simulink model "ctrl_typeBp"  (R2016b)
settings: Solver=ode45  StartTime=0.0  StopTime=10.0  RelTol=1e-3  EnableMultiTasking=on
undefined symbols (not defined in the file): Act_Mat_BF, Act_Mat_BR, Act_Mat_IM, Act_Mat_IR, Act_Mat_RM, Act_Mat_TM, gain_act_GASBF, gain_act_GASSF, gain_act_LBF, gain_act_LIM, gain_act_LTM, gain_act_PBF, gain_act_PIM, gain_act_PTM, gain_act_RBF, gain_act_RIM, gain_act_TBF, gain_act_TIM, gain_act_VBF, gain_act_VIM, gain_act_YBF, gain_act_YIM, gain_act_YTM, gain_GASBF, gain_GASSF, gain_global_LIM, gain_global_LTM, gain_LBF, gain_LIM, gain_oplev_LTM, gain_oplev_PIM, gain_oplev_PTM, gain_oplev_YIM, gain_oplev_YTM, gain_PBF, gain_PIM, gain_RBF, gain_RIM, gain_TBF, gain_TIM, gain_VBF, gain_VIM, gain_YBF, gain_YIM, Sens_Mat_OL, sys1
libraries: cstblocks x21, simulink x3
settings Model: Creator=TAMA Project  LastModifiedBy=miyo
settings DataIOCC: LimitDataPoints=on  SaveFormat=Array  SignalLoggingSaveFormat=ModelDataLogs
settings OptimizationCC: DefaultParameterBehavior=Inlined  BufferReuse=off  ExpressionDepthLimit=2147483647  LifeSpan=inf
settings DebuggingCC: UnderspecifiedInitializationDetection=Classic  MergeDetectMultiDrivingBlocksExec=none  FcnCallInpInsideContextMsg=warning  StateNameClashWarn=warning  InitInArrayFormatMsg=none  SFUnexpectedBacktrackingDiag=warning  SFNoUnconditionalDefaultTransitionDiag=warning  SFExecutionAtInitializationDiag=none
settings HardwareCC: ProdBitPerPointer=32  ProdBitPerSizeT=32  ProdBitPerPtrDiffT=32  ProdLargestAtomicFloat=None  ProdIntDivRoundTo=Undefined  ProdEndianess=Unspecified  ProdWordSize=32  ProdHWDeviceType=32-bit Generic
settings ModelReferenceCC: PropagateSignalLabelsOutOfModel=off
settings GRTTargetCC: TargetLangStandard=C89/C90 (ANSI)  GeneratePreprocessorConditionals=Disable all  CombineOutputUpdateFcns=off  GRTInterface=on
settings ConfigComp: CovMetricSettings=dw  CovHtmlReporting=on  CovSaveCumulativeToWorkspaceVar=on  CovSaveSingleToWorkspaceVar=on  CovExternalEMLEnable=off  CovSFcnEnable=off

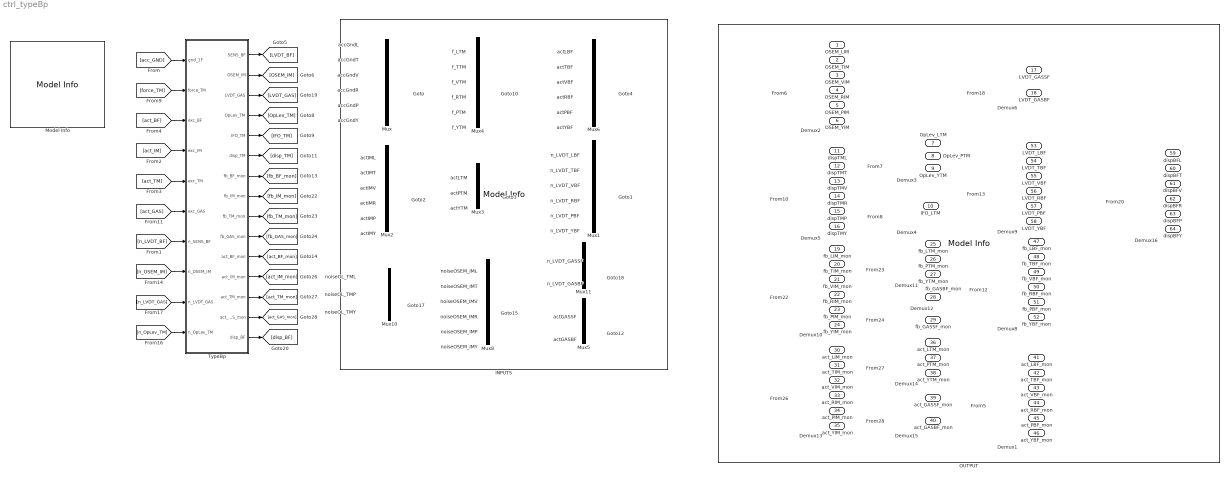
== system ctrl_typeBp ==
  accGndL : Inport
  accGndT : Inport  Port=2
  accGndV : Inport  Port=3
  accGndR : Inport  Port=4
  accGndP : Inport  Port=5
  accGndY : Inport  Port=6
  actIML : Inport  Port=7
  actIMT : Inport  Port=8
  actIMV : Inport  Port=9
  actIMR : Inport  Port=10
  actIMP : Inport  Port=11
  actIMY : Inport  Port=12
  actLTM : Inport  Port=13
  actPTM : Inport  Port=14
  actYTM : Inport  Port=15
  f_LTM : Inport  Port=16
  f_TTM : Inport  Port=17
  f_VTM : Inport  Port=18
  f_RTM : Inport  Port=19
  f_PTM : Inport  Port=20
  f_YTM : Inport  Port=21
  actGASSF : Inport  Port=22
  actGASBF : Inport  Port=23
  noiseOSEM_IML : Inport  Port=24
  noiseOSEM_IMT : Inport  Port=25
  noiseOSEM_IMV : Inport  Port=26
  noiseOSEM_IMR : Inport  Port=27
  noiseOSEM_IMP : Inport  Port=28
  noiseOSEM_IMY : Inport  Port=29
  noiseOL_TML : Inport  Port=30
  noiseOL_TMP : Inport  Port=31
  noiseOL_TMY : Inport  Port=32
  n_LVDT_GASSF : Inport  Port=33
  n_LVDT_GASBF : Inport  Port=34
  n_LVDT_LBF : Inport  Port=35
  n_LVDT_TBF : Inport  Port=36
  n_LVDT_VBF : Inport  Port=37
  n_LVDT_RBF : Inport  Port=38
  n_LVDT_PBF : Inport  Port=39
  n_LVDT_YBF : Inport  Port=40
  actLBF : Inport  Port=41
  actTBF : Inport  Port=42
  actVBF : Inport  Port=43
  actRBF : Inport  Port=44
  actPBF : Inport  Port=45
  actYBF : Inport  Port=46
  Demux{1..2,5,8..10,13,16} (8 alike) : Demux  Outputs=6
  Demux11 : Demux  Outputs=3
  Demux12 : Demux  Outputs=2
  Demux14 : Demux  Outputs=3
  Demux15 : Demux  Outputs=2
  Demux3 : Demux  Outputs=3
  Demux4 : Demux  Outputs=1
  Demux6 : Demux  Outputs=2
  INPUTS : simulink/Model-Wide Utilities/Model Info  BlockCM=none  Frame=on  DisplayStringWithTags=_  HorizontalTextAlignment=Left  LeftAlignmentValue=0.02  SourceBlockDiagram=ctrl_typeBp  TagMaxNumber=20
  Model Info : simulink/Model-Wide Utilities/Model Info  BlockCM=none  Frame=on  DisplayStringWithTags=|  HorizontalTextAlignment=Left  LeftAlignmentValue=0.02  SourceBlockDiagram=ctrl_typeBp  TagMaxNumber=20
      | [MODEL INFORMATION]
      | 
      | ModelName: %<ModelName>
      | LastUpdate : %<LastModificationDate>
      | 
      | TypeBp control model
  Mux{,1..2,4,6,8} (6 alike) : Mux  Inputs=6
  Mux10 : Mux  Inputs=3
  Mux11 : Mux  Inputs=2
  Mux3 : Mux  Inputs=3
  Mux5 : Mux  Inputs=2
  OUTPUT : simulink/Model-Wide Utilities/Model Info  BlockCM=none  Frame=on  DisplayStringWithTags=_  HorizontalTextAlignment=Left  LeftAlignmentValue=0.02  SourceBlockDiagram=ctrl_typeBp  TagMaxNumber=20
  TypeBp : Subsystem
  OSEM_LIM : Outport
  OSEM_TIM : Outport  Port=2
  OSEM_VIM : Outport  Port=3
  OSEM_RIM : Outport  Port=4
  OSEM_PIM : Outport  Port=5
  OSEM_YIM : Outport  Port=6
  OpLev_LTM : Outport  Port=7
  OpLev_PTM : Outport  Port=8
  OpLev_YTM : Outport  Port=9
  IFO_LTM : Outport  Port=10
  dispTML : Outport  Port=11
  dispTMT : Outport  Port=12
  dispTMV : Outport  Port=13
  dispTMR : Outport  Port=14
  dispTMP : Outport  Port=15
  dispTMY : Outport  Port=16
  LVDT_GASSF : Outport  Port=17
  LVDT_GASBF : Outport  Port=18
  fb_LIM_mon : Outport  Port=19
  fb_TIM_mon : Outport  Port=20
  fb_VIM_mon : Outport  Port=21
  fb_RIM_mon : Outport  Port=22
  fb_PIM_mon : Outport  Port=23
  fb_YIM_mon : Outport  Port=24
  fb_LTM_mon : Outport  Port=25
  fb_PTM_mon : Outport  Port=26
  fb_YTM_mon : Outport  Port=27
  fb_GASBF_mon : Outport  Port=28
  fb_GASSF_mon : Outport  Port=29
  act_LIM_mon : Outport  Port=30
  act_TIM_mon : Outport  Port=31
  act_VIM_mon : Outport  Port=32
  act_RIM_mon : Outport  Port=33
  act_PIM_mon : Outport  Port=34
  act_YIM_mon : Outport  Port=35
  act_LTM_mon : Outport  Port=36
  act_PTM_mon : Outport  Port=37
  act_YTM_mon : Outport  Port=38
  act_GASSF_mon : Outport  Port=39
  act_GASBF_mon : Outport  Port=40
  act_LBF_mon : Outport  Port=41
  act_TBF_mon : Outport  Port=42
  act_VBF_mon : Outport  Port=43
  act_RBF_mon : Outport  Port=44
  act_PBF_mon : Outport  Port=45
  act_YBF_mon : Outport  Port=46
  fb_LBF_mon : Outport  Port=47
  fb_TBF_mon : Outport  Port=48
  fb_VBF_mon : Outport  Port=49
  fb_RBF_mon : Outport  Port=50
  fb_PBF_mon : Outport  Port=51
  fb_YBF_mon : Outport  Port=52
  LVDT_LBF : Outport  Port=53
  LVDT_TBF : Outport  Port=54
  LVDT_VBF : Outport  Port=55
  LVDT_RBF : Outport  Port=56
  LVDT_PBF : Outport  Port=57
  LVDT_YBF : Outport  Port=58
  dispBFL : Outport  Port=59
  dispBFT : Outport  Port=60
  dispBFV : Outport  Port=61
  dispBFR : Outport  Port=62
  dispBFP : Outport  Port=63
  dispBFY : Outport  Port=64
  wires:
  accGndL/1 -> Mux/1
  accGndT/1 -> Mux/2
  accGndV/1 -> Mux/3
  accGndR/1 -> Mux/4
  accGndP/1 -> Mux/5
  accGndY/1 -> Mux/6
  Mux/1 -> [acc_GND]
  actIML/1 -> Mux2/1
  actIMT/1 -> Mux2/2
  actIMV/1 -> Mux2/3
  actIMR/1 -> Mux2/4
  actIMP/1 -> Mux2/5
  actIMY/1 -> Mux2/6
  Mux2/1 -> [act_IM]
  actLTM/1 -> Mux3/1
  actPTM/1 -> Mux3/2
  actYTM/1 -> Mux3/3
  Mux3/1 -> [act_TM]
  [OSEM_IM] -> Demux2/1
  Demux2/1 -> OSEM_LIM/1
  Demux2/2 -> OSEM_TIM/1
  Demux2/3 -> OSEM_VIM/1
  Demux2/4 -> OSEM_RIM/1
  Demux2/5 -> OSEM_PIM/1
  Demux2/6 -> OSEM_YIM/1
  [IFO_TM] -> Demux4/1
  Demux4/1 -> IFO_LTM/1
  f_LTM/1 -> Mux4/1
  f_TTM/1 -> Mux4/2
  f_VTM/1 -> Mux4/3
  Mux4/1 -> [force_TM]
  f_YTM/1 -> Mux4/6
  f_PTM/1 -> Mux4/5
  f_RTM/1 -> Mux4/4
  [disp_TM] -> Demux5/1
  Demux5/1 -> dispTML/1
  Demux5/2 -> dispTMT/1
  Demux5/3 -> dispTMV/1
  Demux5/4 -> dispTMR/1
  Demux5/5 -> dispTMP/1
  Demux5/6 -> dispTMY/1
  actGASBF/1 -> Mux5/2
  Mux5/1 -> [act_GAS]
  noiseOSEM_IML/1 -> Mux8/1
  noiseOSEM_IMT/1 -> Mux8/2
  noiseOSEM_IMV/1 -> Mux8/3
  noiseOSEM_IMR/1 -> Mux8/4
  noiseOSEM_IMP/1 -> Mux8/5
  noiseOSEM_IMY/1 -> Mux8/6
  Mux8/1 -> [n_OSEM_IM]
  Mux10/1 -> [n_OpLev_TM]
  n_LVDT_GASBF/1 -> Mux11/2
  Mux11/1 -> [n_LVDT_GAS]
  [LVDT_GAS] -> Demux6/1
  n_LVDT_GASSF/1 -> Mux11/1
  Demux6/1 -> LVDT_GASSF/1
  Demux6/2 -> LVDT_GASBF/1
  actGASSF/1 -> Mux5/1
  [fb_IM_mon] -> Demux10/1
  Demux10/1 -> fb_LIM_mon/1
  Demux10/2 -> fb_TIM_mon/1
  Demux10/3 -> fb_VIM_mon/1
  Demux10/4 -> fb_RIM_mon/1
  Demux10/5 -> fb_PIM_mon/1
  Demux10/6 -> fb_YIM_mon/1
  [fb_TM_mon] -> Demux11/1
  Demux11/1 -> fb_LTM_mon/1
  Demux11/2 -> fb_PTM_mon/1
  Demux11/3 -> fb_YTM_mon/1
  [fb_GAS_mon] -> Demux12/1
  Demux12/1 -> fb_GASBF_mon/1
  Demux12/2 -> fb_GASSF_mon/1
  [act_IM_mon] -> Demux13/1
  Demux13/1 -> act_LIM_mon/1
  Demux13/2 -> act_TIM_mon/1
  Demux13/3 -> act_VIM_mon/1
  Demux13/4 -> act_RIM_mon/1
  Demux13/5 -> act_PIM_mon/1
  Demux13/6 -> act_YIM_mon/1
  [act_TM_mon] -> Demux14/1
  Demux14/1 -> act_LTM_mon/1
  Demux14/2 -> act_PTM_mon/1
  Demux14/3 -> act_YTM_mon/1
  [act_GAS_mon] -> Demux15/1
  Demux15/1 -> act_GASSF_mon/1
  Demux15/2 -> act_GASBF_mon/1
  n_LVDT_TBF/1 -> Mux1/2
  Mux1/1 -> [n_LVDT_BF]
  n_LVDT_LBF/1 -> Mux1/1
  n_LVDT_VBF/1 -> Mux1/3
  actTBF/1 -> Mux6/2
  Mux6/1 -> [act_BF]
  actLBF/1 -> Mux6/1
  actVBF/1 -> Mux6/3
  [act_BF_mon] -> Demux1/1
  Demux1/1 -> act_LBF_mon/1
  Demux1/2 -> act_TBF_mon/1
  Demux1/3 -> act_VBF_mon/1
  [fb_BF_mon] -> Demux8/1
  Demux8/1 -> fb_LBF_mon/1
  Demux8/2 -> fb_TBF_mon/1
  Demux8/3 -> fb_VBF_mon/1
  [LVDT_BF] -> Demux9/1
  Demux9/1 -> LVDT_LBF/1
  Demux9/2 -> LVDT_TBF/1
  Demux9/3 -> LVDT_VBF/1
  [acc_GND] -> TypeBp/1(gnd_1F)
  [force_TM] -> TypeBp/2(force_TM)
  [act_BF] -> TypeBp/3(exc_BF)
  [act_IM] -> TypeBp/4(exc_IM)
  [act_TM] -> TypeBp/5(exc_TM)
  [act_GAS] -> TypeBp/6(exc_GAS)
  [n_LVDT_BF] -> TypeBp/7(n_SENS_BF)
  [n_OSEM_IM] -> TypeBp/8(n_OSEM_IM)
  [n_LVDT_GAS] -> TypeBp/9(n_LVDT_GAS)
  [n_OpLev_TM] -> TypeBp/10(n_OpLev_TM)
  TypeBp/1(SENS_BF) -> [LVDT_BF]
  TypeBp/2(OSEM_IM) -> [OSEM_IM]
  TypeBp/3(LVDT_GAS) -> [LVDT_GAS]
  TypeBp/4(OpLev_TM) -> [OpLev_TM]
  TypeBp/5(IFO_TM) -> [IFO_TM]
  TypeBp/6(disp_TM) -> [disp_TM]
  TypeBp/7(fb_BF_mon) -> [fb_BF_mon]
  TypeBp/8(fb_IM_mon) -> [fb_IM_mon]
  TypeBp/9(fb_TM_mon) -> [fb_TM_mon]
  TypeBp/10(fb_GAS_mon) -> [fb_GAS_mon]
  TypeBp/12(act_IM_mon) -> [act_IM_mon]
  TypeBp/14(act_GAS_mon) -> [act_GAS_mon]
  actRBF/1 -> Mux6/4
  actPBF/1 -> Mux6/5
  actYBF/1 -> Mux6/6
  n_LVDT_RBF/1 -> Mux1/4
  n_LVDT_PBF/1 -> Mux1/5
  n_LVDT_YBF/1 -> Mux1/6
  Demux9/4 -> LVDT_RBF/1
  Demux9/5 -> LVDT_PBF/1
  Demux9/6 -> LVDT_YBF/1
  Demux8/4 -> fb_RBF_mon/1
  Demux8/5 -> fb_PBF_mon/1
  Demux8/6 -> fb_YBF_mon/1
  Demux1/4 -> act_RBF_mon/1
  Demux1/5 -> act_PBF_mon/1
  Demux1/6 -> act_YBF_mon/1
  TypeBp/15(disp_BF) -> [disp_BF]
  [disp_BF] -> Demux16/1
  Demux16/1 -> dispBFL/1
  Demux16/2 -> dispBFT/1
  Demux16/3 -> dispBFV/1
  Demux16/4 -> dispBFR/1
  Demux16/5 -> dispBFP/1
  Demux16/6 -> dispBFY/1
  TypeBp/11(act_BF_mon) -> [act_BF_mon]
  TypeBp/13(act_TM_mon) -> [act_TM_mon]
  noiseOL_TMP/1 -> Mux10/2
  noiseOL_TML/1 -> Mux10/1
  noiseOL_TMY/1 -> Mux10/3
  Demux3/2 -> OpLev_PTM/1
  Demux3/3 -> OpLev_YTM/1
  Demux3/1 -> OpLev_LTM/1
  [OpLev_TM] -> Demux3/1

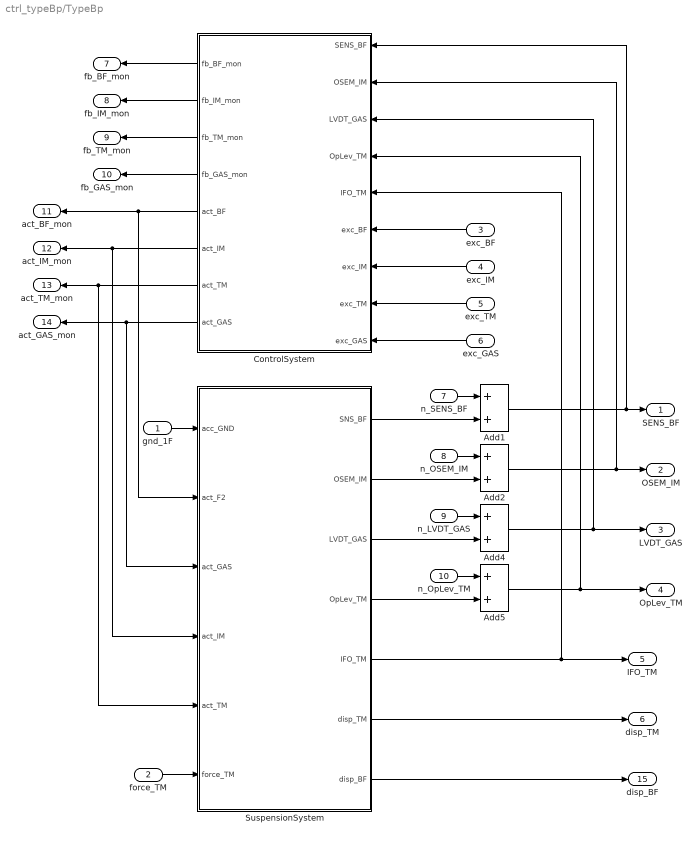
== system ctrl_typeBp/TypeBp ==
  gnd_1F : Inport
  force_TM : Inport  Port=2
  exc_BF : Inport  Port=3
  exc_IM : Inport  Port=4
  exc_TM : Inport  Port=5
  exc_GAS : Inport  Port=6
  n_SENS_BF : Inport  Port=7
  n_OSEM_IM : Inport  Port=8
  n_LVDT_GAS : Inport  Port=9
  n_OpLev_TM : Inport  Port=10
  Add{1..2,4..5} (4 alike) : Sum
  ControlSystem : Subsystem
  SuspensionSystem : Subsystem
  SENS_BF : Outport
  OSEM_IM : Outport  Port=2
  LVDT_GAS : Outport  Port=3
  OpLev_TM : Outport  Port=4
  IFO_TM : Outport  Port=5
  disp_TM : Outport  Port=6
  fb_BF_mon : Outport  Port=7
  fb_IM_mon : Outport  Port=8
  fb_TM_mon : Outport  Port=9
  fb_GAS_mon : Outport  Port=10
  act_BF_mon : Outport  Port=11
  act_IM_mon : Outport  Port=12
  act_TM_mon : Outport  Port=13
  act_GAS_mon : Outport  Port=14
  disp_BF : Outport  Port=15
  wires:
  gnd_1F/1 -> SuspensionSystem/1(acc_GND)
  force_TM/1 -> SuspensionSystem/6(force_TM)
  SuspensionSystem/6(disp_TM) -> disp_TM/1
  SuspensionSystem/2(OSEM_IM) -> Add2/2
  n_OSEM_IM/1 -> Add2/1
  SuspensionSystem/5(IFO_TM) -> IFO_TM/1, ControlSystem/5(IFO_TM)
  Add2/1 -> ControlSystem/2(OSEM_IM), OSEM_IM/1
  n_LVDT_GAS/1 -> Add4/1
  SuspensionSystem/3(LVDT_GAS) -> Add4/2
  n_OpLev_TM/1 -> Add5/1
  SuspensionSystem/4(OpLev_TM) -> Add5/2
  Add4/1 -> ControlSystem/3(LVDT_GAS), LVDT_GAS/1
  Add5/1 -> ControlSystem/4(OpLev_TM), OpLev_TM/1
  Add1/1 -> ControlSystem/1(SENS_BF), SENS_BF/1
  SuspensionSystem/1(SNS_BF) -> Add1/2
  n_SENS_BF/1 -> Add1/1
  exc_BF/1 -> ControlSystem/6(exc_BF)
  exc_IM/1 -> ControlSystem/7(exc_IM)
  exc_TM/1 -> ControlSystem/8(exc_TM)
  exc_GAS/1 -> ControlSystem/9(exc_GAS)
  ControlSystem/1(fb_BF_mon) -> fb_BF_mon/1
  ControlSystem/2(fb_IM_mon) -> fb_IM_mon/1
  ControlSystem/3(fb_TM_mon) -> fb_TM_mon/1
  ControlSystem/4(fb_GAS_mon) -> fb_GAS_mon/1
  ControlSystem/5(act_BF) -> act_BF_mon/1, SuspensionSystem/2(act_F2)
  ControlSystem/7(act_TM) -> act_TM_mon/1, SuspensionSystem/5(act_TM)
  ControlSystem/8(act_GAS) -> act_GAS_mon/1, SuspensionSystem/3(act_GAS)
  ControlSystem/6(act_IM) -> act_IM_mon/1, SuspensionSystem/4(act_IM)
  SuspensionSystem/7(disp_BF) -> disp_BF/1

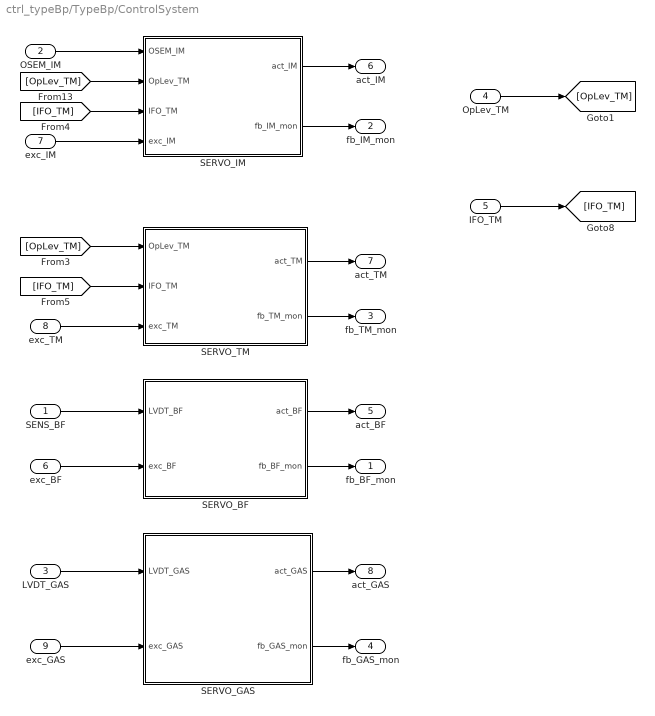
== system ctrl_typeBp/TypeBp/ControlSystem ==
  SENS_BF : Inport
  OSEM_IM : Inport  Port=2
  LVDT_GAS : Inport  Port=3
  OpLev_TM : Inport  Port=4
  IFO_TM : Inport  Port=5
  exc_BF : Inport  Port=6
  exc_IM : Inport  Port=7
  exc_TM : Inport  Port=8
  exc_GAS : Inport  Port=9
  SERVO_BF : Subsystem
  SERVO_GAS : Subsystem
  SERVO_IM : Subsystem
  SERVO_TM : Subsystem
  fb_BF_mon : Outport
  fb_IM_mon : Outport  Port=2
  fb_TM_mon : Outport  Port=3
  fb_GAS_mon : Outport  Port=4
  act_BF : Outport  Port=5
  act_IM : Outport  Port=6
  act_TM : Outport  Port=7
  act_GAS : Outport  Port=8
  wires:
  IFO_TM/1 -> [IFO_TM]
  OpLev_TM/1 -> [OpLev_TM]
  SERVO_IM/1(act_IM) -> act_IM/1
  OSEM_IM/1 -> SERVO_IM/1(OSEM_IM)
  SERVO_TM/1(act_TM) -> act_TM/1
  [OpLev_TM] -> SERVO_IM/2(OpLev_TM)
  [OpLev_TM] -> SERVO_TM/1(OpLev_TM)
  [IFO_TM] -> SERVO_IM/3(IFO_TM)
  [IFO_TM] -> SERVO_TM/2(IFO_TM)
  exc_IM/1 -> SERVO_IM/4(exc_IM)
  exc_TM/1 -> SERVO_TM/3(exc_TM)
  SERVO_IM/2(fb_IM_mon) -> fb_IM_mon/1
  SERVO_TM/2(fb_TM_mon) -> fb_TM_mon/1
  exc_GAS/1 -> SERVO_GAS/2(exc_GAS)
  SERVO_GAS/2(fb_GAS_mon) -> fb_GAS_mon/1
  LVDT_GAS/1 -> SERVO_GAS/1(LVDT_GAS)
  SERVO_GAS/1(act_GAS) -> act_GAS/1
  SENS_BF/1 -> SERVO_BF/1(LVDT_BF)
  SERVO_BF/1(act_BF) -> act_BF/1
  exc_BF/1 -> SERVO_BF/2(exc_BF)
  SERVO_BF/2(fb_BF_mon) -> fb_BF_mon/1

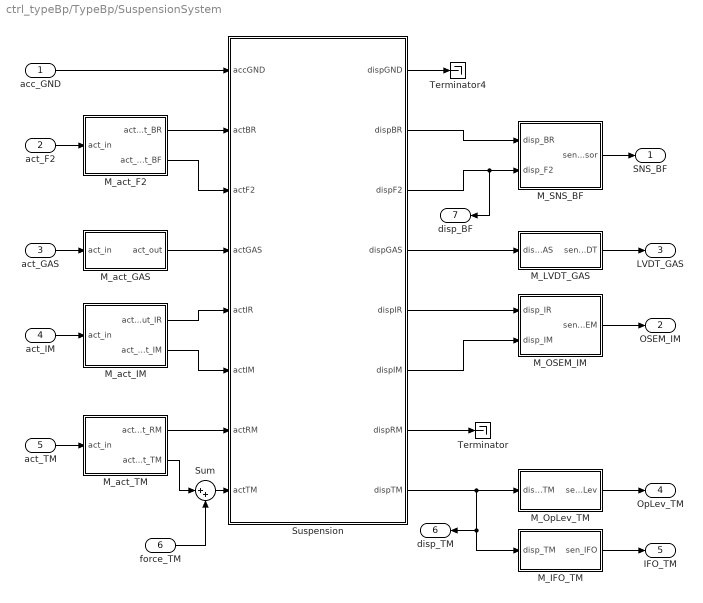
== system ctrl_typeBp/TypeBp/SuspensionSystem ==
  acc_GND : Inport
  act_F2 : Inport  Port=2
  act_GAS : Inport  Port=3
  act_IM : Inport  Port=4
  act_TM : Inport  Port=5
  force_TM : Inport  Port=6
  M_IFO_TM : Subsystem
  M_LVDT_GAS : Subsystem
  M_OSEM_IM : Subsystem
  M_OpLev_TM : Subsystem
  M_SNS_BF : Subsystem
  M_act_F2 : Subsystem
  M_act_GAS : Subsystem
  M_act_IM : Subsystem
  M_act_TM : Subsystem
  Sum : Sum  Inputs=|++
  Suspension : Subsystem
  Terminator : Terminator
  Terminator4 : Terminator
  SNS_BF : Outport
  OSEM_IM : Outport  Port=2
  LVDT_GAS : Outport  Port=3
  OpLev_TM : Outport  Port=4
  IFO_TM : Outport  Port=5
  disp_TM : Outport  Port=6
  disp_BF : Outport  Port=7
  wires:
  act_IM/1 -> M_act_IM/1(act_in)
  act_TM/1 -> M_act_TM/1(act_in)
  act_GAS/1 -> M_act_GAS/1(act_in)
  M_OSEM_IM/1(sen_OSEM) -> OSEM_IM/1
  M_LVDT_GAS/1(sen_LVDT) -> LVDT_GAS/1
  M_IFO_TM/1(sen_IFO) -> IFO_TM/1
  M_OpLev_TM/1(sen_OpLev) -> OpLev_TM/1
  act_F2/1 -> M_act_F2/1(act_in)
  acc_GND/1 -> Suspension/1(accGND)
  M_act_F2/1(act_out_BR) -> Suspension/2(actBR)
  M_act_F2/2(act_out_BF) -> Suspension/3(actF2)
  M_act_GAS/1(act_out) -> Suspension/4(actGAS)
  M_act_IM/1(act_out_IR) -> Suspension/5(actIR)
  M_act_IM/2(act_out_IM) -> Suspension/6(actIM)
  M_act_TM/1(act_out_RM) -> Suspension/7(actRM)
  M_act_TM/2(act_out_TM) -> Sum/1
  force_TM/1 -> Sum/2
  Sum/1 -> Suspension/8(actTM)
  M_SNS_BF/1(sen_F2sensor) -> SNS_BF/1
  Suspension/2(dispBR) -> M_SNS_BF/1(disp_BR)
  Suspension/3(dispF2) -> disp_BF/1, M_SNS_BF/2(disp_F2)
  Suspension/1(dispGND) -> Terminator4/1
  Suspension/4(dispGAS) -> M_LVDT_GAS/1(disp_GAS)
  Suspension/5(dispIR) -> M_OSEM_IM/1(disp_IR)
  Suspension/6(dispIM) -> M_OSEM_IM/2(disp_IM)
  Suspension/8(dispTM) -> M_IFO_TM/1(disp_TM), disp_TM/1, M_OpLev_TM/1(disp_TM)
  Suspension/7(dispRM) -> Terminator/1

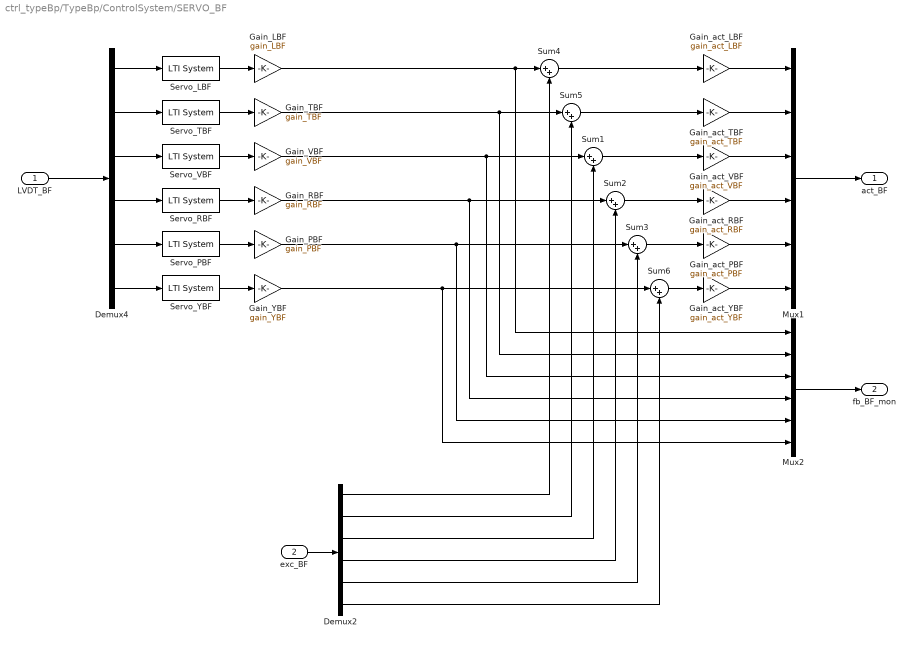
== system ctrl_typeBp/TypeBp/ControlSystem/SERVO_BF ==
  LVDT_BF : Inport
  exc_BF : Inport  Port=2
  Demux2 : Demux  Outputs=6
  Demux4 : Demux  Outputs=6
  Gain_LBF : Gain  Gain=gain_LBF
  Gain_PBF : Gain  Gain=gain_PBF
  Gain_RBF : Gain  Gain=gain_RBF
  Gain_TBF : Gain  Gain=gain_TBF
  Gain_VBF : Gain  Gain=gain_VBF
  Gain_YBF : Gain  Gain=gain_YBF
  Gain_act_LBF : Gain  Gain=gain_act_LBF
  Gain_act_PBF : Gain  Gain=gain_act_PBF
  Gain_act_RBF : Gain  Gain=gain_act_RBF
  Gain_act_TBF : Gain  Gain=gain_act_TBF
  Gain_act_VBF : Gain  Gain=gain_act_VBF
  Gain_act_YBF : Gain  Gain=gain_act_YBF
  Mux1 : Mux  Inputs=6
  Mux2 : Mux  Inputs=6
  Servo_LBF : cstblocks/LTI System  sys=servo_LBF  IC=[]
  Servo_PBF : cstblocks/LTI System  sys=servo_PBF  IC=[]
  Servo_RBF : cstblocks/LTI System  sys=servo_RBF  IC=[]
  Servo_TBF : cstblocks/LTI System  sys=servo_TBF  IC=[]
  Servo_VBF : cstblocks/LTI System  sys=servo_VBF  IC=[]
  Servo_YBF : cstblocks/LTI System  sys=servo_YBF  IC=[]
  Sum{1..6} (6 alike) : Sum  Inputs=|++
  act_BF : Outport
  fb_BF_mon : Outport  Port=2
  wires:
  Demux4/1 -> Servo_LBF/1
  Demux4/2 -> Servo_TBF/1
  Servo_LBF/1 -> Gain_LBF/1
  Servo_TBF/1 -> Gain_TBF/1
  LVDT_BF/1 -> Demux4/1
  Mux1/1 -> act_BF/1
  Gain_act_LBF/1 -> Mux1/1
  Gain_act_TBF/1 -> Mux1/2
  Gain_LBF/1 -> Mux2/1, Sum4/1
  Sum4/1 -> Gain_act_LBF/1
  Gain_TBF/1 -> Mux2/2, Sum5/1
  Sum5/1 -> Gain_act_TBF/1
  exc_BF/1 -> Demux2/1
  Mux2/1 -> fb_BF_mon/1
  Demux4/3 -> Servo_VBF/1
  Servo_VBF/1 -> Gain_VBF/1
  Gain_act_VBF/1 -> Mux1/3
  Sum1/1 -> Gain_act_VBF/1
  Gain_VBF/1 -> Mux2/3, Sum1/1
  Demux2/1 -> Sum4/2
  Demux2/2 -> Sum5/2
  Demux2/3 -> Sum1/2
  Demux4/4 -> Servo_RBF/1
  Servo_RBF/1 -> Gain_RBF/1
  Gain_act_RBF/1 -> Mux1/4
  Gain_RBF/1 -> Mux2/4, Sum2/1
  Sum2/1 -> Gain_act_RBF/1
  Demux4/5 -> Servo_PBF/1
  Servo_PBF/1 -> Gain_PBF/1
  Gain_act_PBF/1 -> Mux1/5
  Gain_PBF/1 -> Mux2/5, Sum3/1
  Sum3/1 -> Gain_act_PBF/1
  Demux4/6 -> Servo_YBF/1
  Servo_YBF/1 -> Gain_YBF/1
  Gain_act_YBF/1 -> Mux1/6
  Gain_YBF/1 -> Mux2/6, Sum6/1
  Sum6/1 -> Gain_act_YBF/1
  Demux2/4 -> Sum2/2
  Demux2/5 -> Sum3/2
  Demux2/6 -> Sum6/2

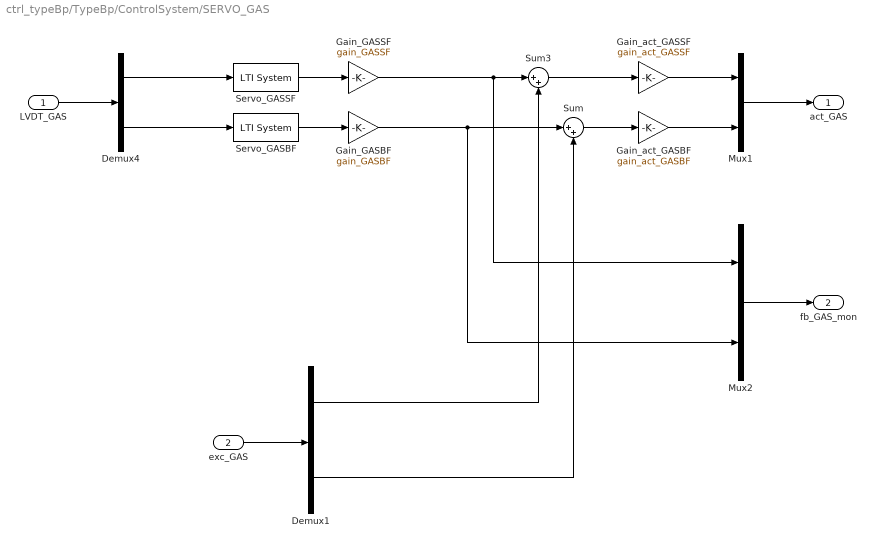
== system ctrl_typeBp/TypeBp/ControlSystem/SERVO_GAS ==
  LVDT_GAS : Inport
  exc_GAS : Inport  Port=2
  Demux1 : Demux  Outputs=2
  Demux4 : Demux  Outputs=2
  Gain_GASBF : Gain  Gain=gain_GASBF
  Gain_GASSF : Gain  Gain=gain_GASSF
  Gain_act_GASBF : Gain  Gain=gain_act_GASBF
  Gain_act_GASSF : Gain  Gain=gain_act_GASSF
  Mux1 : Mux  Inputs=2
  Mux2 : Mux  Inputs=2
  Servo_GASBF : cstblocks/LTI System  sys=servo_GASBF  IC=[]
  Servo_GASSF : cstblocks/LTI System  sys=servo_GASSF  IC=[]
  Sum : Sum  Inputs=|++
  Sum3 : Sum  Inputs=|++
  act_GAS : Outport
  fb_GAS_mon : Outport  Port=2
  wires:
  Servo_GASSF/1 -> Gain_GASSF/1
  Servo_GASBF/1 -> Gain_GASBF/1
  LVDT_GAS/1 -> Demux4/1
  Mux1/1 -> act_GAS/1
  exc_GAS/1 -> Demux1/1
  Gain_GASSF/1 -> Sum3/1, Mux2/1
  Sum3/1 -> Gain_act_GASSF/1
  Gain_GASBF/1 -> Sum/1, Mux2/2
  Sum/1 -> Gain_act_GASBF/1
  Mux2/1 -> fb_GAS_mon/1
  Demux4/1 -> Servo_GASSF/1
  Demux4/2 -> Servo_GASBF/1
  Gain_act_GASSF/1 -> Mux1/1
  Gain_act_GASBF/1 -> Mux1/2
  Demux1/1 -> Sum3/2
  Demux1/2 -> Sum/2

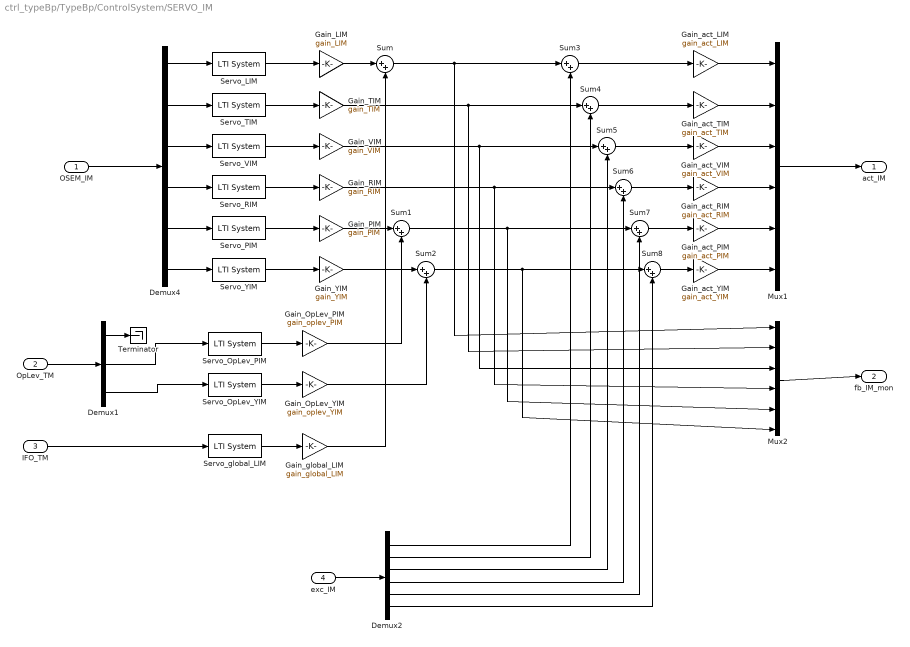
== system ctrl_typeBp/TypeBp/ControlSystem/SERVO_IM ==
  OSEM_IM : Inport
  OpLev_TM : Inport  Port=2
  IFO_TM : Inport  Port=3
  exc_IM : Inport  Port=4
  Demux1 : Demux  Outputs=3
  Demux2 : Demux  Outputs=6
  Demux4 : Demux  Outputs=6
  Gain_LIM : Gain  Gain=gain_LIM
  Gain_OpLev_PIM : Gain  Gain=gain_oplev_PIM
  Gain_OpLev_YIM : Gain  Gain=gain_oplev_YIM
  Gain_PIM : Gain  Gain=gain_PIM
  Gain_RIM : Gain  Gain=gain_RIM
  Gain_TIM : Gain  Gain=gain_TIM
  Gain_VIM : Gain  Gain=gain_VIM
  Gain_YIM : Gain  Gain=gain_YIM
  Gain_act_LIM : Gain  Gain=gain_act_LIM
  Gain_act_PIM : Gain  Gain=gain_act_PIM
  Gain_act_RIM : Gain  Gain=gain_act_RIM
  Gain_act_TIM : Gain  Gain=gain_act_TIM
  Gain_act_VIM : Gain  Gain=gain_act_VIM
  Gain_act_YIM : Gain  Gain=gain_act_YIM
  Gain_global_LIM : Gain  Gain=gain_global_LIM
  Mux1 : Mux  Inputs=6
  Mux2 : Mux  Inputs=6
  Servo_LIM : cstblocks/LTI System  sys=servo_LIM  IC=[]
  Servo_OpLev_PIM : cstblocks/LTI System  sys=servo_oplev_PIM  IC=[]
  Servo_OpLev_YIM : cstblocks/LTI System  sys=servo_oplev_YIM  IC=[]
  Servo_PIM : cstblocks/LTI System  sys=servo_PIM  IC=[]
  Servo_RIM : cstblocks/LTI System  sys=servo_RIM  IC=[]
  Servo_TIM : cstblocks/LTI System  sys=servo_TIM  IC=[]
  Servo_VIM : cstblocks/LTI System  sys=servo_VIM  IC=[]
  Servo_YIM : cstblocks/LTI System  sys=servo_YIM  IC=[]
  Servo_global_LIM : cstblocks/LTI System  sys=servo_global_LIM  IC=[]
  Sum{,1..8} (9 alike) : Sum  Inputs=|++
  Terminator : Terminator
  act_IM : Outport
  fb_IM_mon : Outport  Port=2
  wires:
  Demux4/1 -> Servo_LIM/1
  Demux4/2 -> Servo_TIM/1
  Demux4/3 -> Servo_VIM/1
  Servo_LIM/1 -> Gain_LIM/1
  Servo_TIM/1 -> Gain_TIM/1
  Servo_VIM/1 -> Gain_VIM/1
  Mux1/1 -> act_IM/1
  Gain_act_LIM/1 -> Mux1/1
  Gain_act_TIM/1 -> Mux1/2
  Gain_act_VIM/1 -> Mux1/3
  OSEM_IM/1 -> Demux4/1
  Servo_RIM/1 -> Gain_RIM/1
  Servo_PIM/1 -> Gain_PIM/1
  Servo_YIM/1 -> Gain_YIM/1
  Demux4/4 -> Servo_RIM/1
  Demux4/5 -> Servo_PIM/1
  Demux4/6 -> Servo_YIM/1
  Gain_act_RIM/1 -> Mux1/4
  Gain_act_PIM/1 -> Mux1/5
  Gain_act_YIM/1 -> Mux1/6
  OpLev_TM/1 -> Demux1/1
  IFO_TM/1 -> Servo_global_LIM/1
  Gain_LIM/1 -> Sum/1
  Servo_global_LIM/1 -> Gain_global_LIM/1
  Gain_PIM/1 -> Sum1/1
  Gain_YIM/1 -> Sum2/1
  Gain_global_LIM/1 -> Sum/2
  Servo_OpLev_PIM/1 -> Gain_OpLev_PIM/1
  Servo_OpLev_YIM/1 -> Gain_OpLev_YIM/1
  Gain_OpLev_PIM/1 -> Sum1/2
  Gain_OpLev_YIM/1 -> Sum2/2
  Sum/1 -> Sum3/1, Mux2/1
  Sum3/1 -> Gain_act_LIM/1
  Gain_TIM/1 -> Mux2/2, Sum4/1
  Sum4/1 -> Gain_act_TIM/1
  Gain_VIM/1 -> Mux2/3, Sum5/1
  Sum5/1 -> Gain_act_VIM/1
  Gain_RIM/1 -> Sum6/1, Mux2/4
  Sum6/1 -> Gain_act_RIM/1
  Sum1/1 -> Sum7/1, Mux2/5
  Sum7/1 -> Gain_act_PIM/1
  Sum2/1 -> Sum8/1, Mux2/6
  Sum8/1 -> Gain_act_YIM/1
  Demux2/1 -> Sum3/2
  Demux2/2 -> Sum4/2
  Demux2/3 -> Sum5/2
  Demux2/4 -> Sum6/2
  Demux2/5 -> Sum7/2
  Demux2/6 -> Sum8/2
  exc_IM/1 -> Demux2/1
  Mux2/1 -> fb_IM_mon/1
  Demux1/2 -> Servo_OpLev_PIM/1
  Demux1/3 -> Servo_OpLev_YIM/1
  Demux1/1 -> Terminator/1

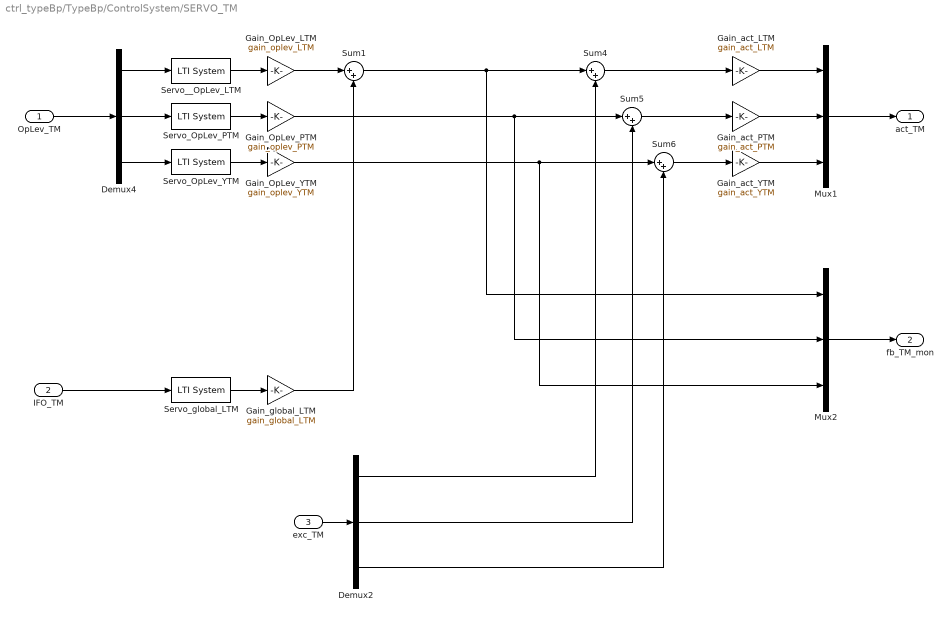
== system ctrl_typeBp/TypeBp/ControlSystem/SERVO_TM ==
  OpLev_TM : Inport
  IFO_TM : Inport  Port=2
  exc_TM : Inport  Port=3
  Demux2 : Demux  Outputs=3
  Demux4 : Demux  Outputs=3
  Gain_OpLev_LTM : Gain  Gain=gain_oplev_LTM
  Gain_OpLev_PTM : Gain  Gain=gain_oplev_PTM
  Gain_OpLev_YTM : Gain  Gain=gain_oplev_YTM
  Gain_act_LTM : Gain  Gain=gain_act_LTM
  Gain_act_PTM : Gain  Gain=gain_act_PTM
  Gain_act_YTM : Gain  Gain=gain_act_YTM
  Gain_global_LTM : Gain  Gain=gain_global_LTM
  Mux1 : Mux  Inputs=3
  Mux2 : Mux  Inputs=3
  Servo_OpLev_PTM : cstblocks/LTI System  sys=servo_oplev_PTM  IC=[]
  Servo_OpLev_YTM : cstblocks/LTI System  sys=servo_oplev_YTM  IC=[]
  Servo__OpLev_LTM : cstblocks/LTI System  sys=servo_oplev_LTM  IC=[]
  Servo_global_LTM : cstblocks/LTI System  sys=servo_global_LTM  IC=[]
  Sum{1,4..6} (4 alike) : Sum  Inputs=|++
  act_TM : Outport
  fb_TM_mon : Outport  Port=2
  wires:
  Demux4/1 -> Servo__OpLev_LTM/1
  Demux4/2 -> Servo_OpLev_PTM/1
  Demux4/3 -> Servo_OpLev_YTM/1
  Servo__OpLev_LTM/1 -> Gain_OpLev_LTM/1
  Servo_OpLev_PTM/1 -> Gain_OpLev_PTM/1
  Servo_OpLev_YTM/1 -> Gain_OpLev_YTM/1
  OpLev_TM/1 -> Demux4/1
  Mux1/1 -> act_TM/1
  IFO_TM/1 -> Servo_global_LTM/1
  Servo_global_LTM/1 -> Gain_global_LTM/1
  Gain_OpLev_LTM/1 -> Sum1/1
  Gain_global_LTM/1 -> Sum1/2
  Gain_act_LTM/1 -> Mux1/1
  Gain_act_PTM/1 -> Mux1/2
  Gain_act_YTM/1 -> Mux1/3
  Sum1/1 -> Mux2/1, Sum4/1
  Sum4/1 -> Gain_act_LTM/1
  Gain_OpLev_PTM/1 -> Mux2/2, Sum5/1
  Sum5/1 -> Gain_act_PTM/1
  Gain_OpLev_YTM/1 -> Mux2/3, Sum6/1
  Sum6/1 -> Gain_act_YTM/1
  exc_TM/1 -> Demux2/1
  Demux2/1 -> Sum4/2
  Demux2/2 -> Sum5/2
  Demux2/3 -> Sum6/2
  Mux2/1 -> fb_TM_mon/1

== system ctrl_typeBp/TypeBp/SuspensionSystem/M_IFO_TM ==
  disp_TM : Inport
  Add2 : Sum  Inputs=++++
  Demux4 : Demux  Outputs=6
  Gain1 : Gain  Gain=1/300
  Gain2 : Gain  Gain=1e-3
  Gain3 : Gain  Gain=1e-3
  Terminator1 : Terminator
  Terminator3 : Terminator
  sen_IFO : Outport
  wires:
  disp_TM/1 -> Demux4/1
  Demux4/4 -> Terminator3/1
  Demux4/3 -> Gain1/1
  Demux4/2 -> Terminator1/1
  Add2/1 -> sen_IFO/1
  Demux4/1 -> Add2/1
  Gain1/1 -> Add2/2
  Demux4/5 -> Gain2/1
  Gain3/1 -> Add2/4
  Gain2/1 -> Add2/3
  Demux4/6 -> Gain3/1

== system ctrl_typeBp/TypeBp/SuspensionSystem/M_LVDT_GAS ==
  disp_GAS : Inport
  Add1 : Sum  Inputs=-+
  Add2 : Sum  Inputs=-+
  Demux4 : Demux  Outputs=3
  Mux3 : Mux  Inputs=2
  sen_LVDT : Outport
  wires:
  disp_GAS/1 -> Demux4/1
  Demux4/1 -> Add2/1
  Demux4/2 -> Add1/1, Add2/2
  Demux4/3 -> Add1/2
  Add2/1 -> Mux3/1
  Add1/1 -> Mux3/2
  Mux3/1 -> sen_LVDT/1

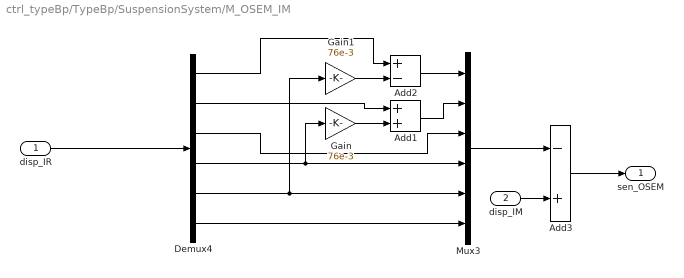
== system ctrl_typeBp/TypeBp/SuspensionSystem/M_OSEM_IM ==
  disp_IR : Inport
  disp_IM : Inport  Port=2
  Add1 : Sum
  Add2 : Sum  Inputs=+-
  Add3 : Sum  Inputs=-+
  Demux4 : Demux  Outputs=6
  Gain : Gain  Gain=76e-3
  Gain1 : Gain  Gain=76e-3
  Mux3 : Mux  Inputs=6
  sen_OSEM : Outport
  wires:
  disp_IM/1 -> Add3/2
  disp_IR/1 -> Demux4/1
  Demux4/6 -> Mux3/6
  Mux3/1 -> Add3/1
  Add3/1 -> sen_OSEM/1
  Demux4/1 -> Add2/1
  Demux4/2 -> Add1/1
  Demux4/3 -> Mux3/3
  Demux4/4 -> Gain/1, Mux3/4
  Demux4/5 -> Gain1/1, Mux3/5
  Gain1/1 -> Add2/2
  Gain/1 -> Add1/2
  Add1/1 -> Mux3/2
  Add2/1 -> Mux3/1

== system ctrl_typeBp/TypeBp/SuspensionSystem/M_OpLev_TM ==
  disp_TM : Inport
  Demux1 : Demux  Outputs=6
  Mux1 : Mux  Inputs=3
  Sens_Mat_OL : Constant  Value=Sens_Mat_OL  VectorParams1D=off
  TM_OpLev_coupling : Product  Multiplication=Matrix(*)
  Terminator4 : Terminator
  Terminator5 : Terminator
  Terminator6 : Terminator
  sen_OpLev : Outport
  wires:
  Demux1/5 -> Mux1/2
  Demux1/6 -> Mux1/3
  Demux1/4 -> Terminator6/1
  Demux1/3 -> Terminator5/1
  Demux1/2 -> Terminator4/1
  Demux1/1 -> Mux1/1
  Mux1/1 -> sen_OpLev/1
  TM_OpLev_coupling/1 -> Demux1/1
  Sens_Mat_OL/1 -> TM_OpLev_coupling/1
  disp_TM/1 -> TM_OpLev_coupling/2

== system ctrl_typeBp/TypeBp/SuspensionSystem/M_SNS_BF ==
  disp_BR : Inport
  disp_F2 : Inport  Port=2
  Add2 : Sum  Inputs=-+
  sen_F2sensor : Outport
  wires:
  Add2/1 -> sen_F2sensor/1
  disp_BR/1 -> Add2/1
  disp_F2/1 -> Add2/2

== system ctrl_typeBp/TypeBp/SuspensionSystem/M_act_F2 ==
  act_in : Inport
  Act_Mat_BF : Constant  Value=Act_Mat_BF  VectorParams1D=off
  Act_Mat_BR : Constant  Value=Act_Mat_BR  VectorParams1D=off
  BF_coupling : Product  Multiplication=Matrix(*)
  BR_coupling : Product  Multiplication=Matrix(*)
  Gain2 : Gain  Gain=-1
  act_out_BR : Outport
  act_out_BF : Outport  Port=2
  wires:
  act_in/1 -> BF_coupling/2, Gain2/1
  Gain2/1 -> BR_coupling/2
  Act_Mat_BR/1 -> BR_coupling/1
  BR_coupling/1 -> act_out_BR/1
  Act_Mat_BF/1 -> BF_coupling/1
  BF_coupling/1 -> act_out_BF/1

== system ctrl_typeBp/TypeBp/SuspensionSystem/M_act_GAS ==
  act_in : Inport
  Add1 : Sum  Inputs=+-
  Demux4 : Demux  Outputs=2
  Mux3 : Mux  Inputs=2
  act_out : Outport
  wires:
  act_in/1 -> Demux4/1
  Mux3/1 -> act_out/1
  Add1/1 -> Mux3/1  "BF"
  Demux4/1 -> Add1/1  "SF"
  Demux4/2 -> Add1/2, Mux3/2  "BF"

== system ctrl_typeBp/TypeBp/SuspensionSystem/M_act_IM ==
  act_in : Inport
  Act_Mat_IM : Constant  Value=Act_Mat_IM  VectorParams1D=off
  Act_Mat_IR : Constant  Value=Act_Mat_IR  VectorParams1D=off
  Gain2 : Gain  Gain=-1
  IM_coupling : Product  Multiplication=Matrix(*)
  IR_coupling : Product  Multiplication=Matrix(*)
  act_out_IR : Outport
  act_out_IM : Outport  Port=2
  wires:
  IR_coupling/1 -> act_out_IR/1
  Act_Mat_IR/1 -> IR_coupling/1
  act_in/1 -> IM_coupling/2, Gain2/1
  Act_Mat_IM/1 -> IM_coupling/1
  IM_coupling/1 -> act_out_IM/1
  Gain2/1 -> IR_coupling/2

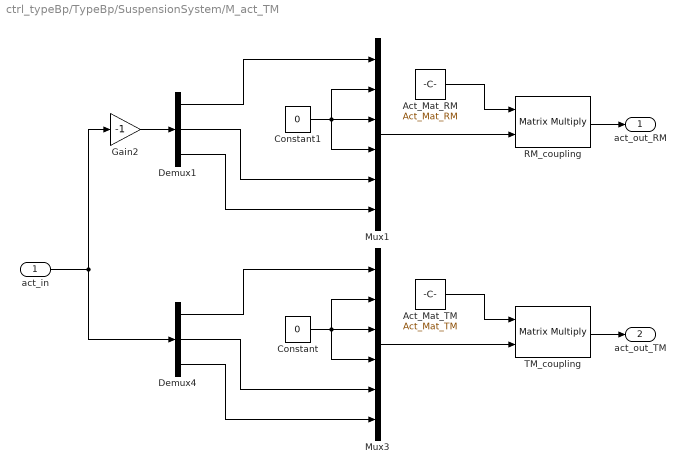
== system ctrl_typeBp/TypeBp/SuspensionSystem/M_act_TM ==
  act_in : Inport
  Act_Mat_RM : Constant  Value=Act_Mat_RM  VectorParams1D=off
  Act_Mat_TM : Constant  Value=Act_Mat_TM  VectorParams1D=off
  Constant : Constant  Value=0
  Constant1 : Constant  Value=0
  Demux1 : Demux  Outputs=3
  Demux4 : Demux  Outputs=3
  Gain2 : Gain  Gain=-1
  Mux1 : Mux  Inputs=6
  Mux3 : Mux  Inputs=6
  RM_coupling : Product  Multiplication=Matrix(*)
  TM_coupling : Product  Multiplication=Matrix(*)
  act_out_RM : Outport
  act_out_TM : Outport  Port=2
  wires:
  Demux4/1 -> Mux3/1
  Demux4/2 -> Mux3/5
  Demux4/3 -> Mux3/6
  Constant/1 -> Mux3/4, Mux3/2, Mux3/3
  Mux3/1 -> TM_coupling/2
  Act_Mat_TM/1 -> TM_coupling/1
  TM_coupling/1 -> act_out_TM/1
  act_in/1 -> Demux4/1, Gain2/1
  Demux1/1 -> Mux1/1
  Demux1/2 -> Mux1/5
  Demux1/3 -> Mux1/6
  Constant1/1 -> Mux1/4, Mux1/2, Mux1/3
  Gain2/1 -> Demux1/1
  Mux1/1 -> RM_coupling/2
  Act_Mat_RM/1 -> RM_coupling/1
  RM_coupling/1 -> act_out_RM/1

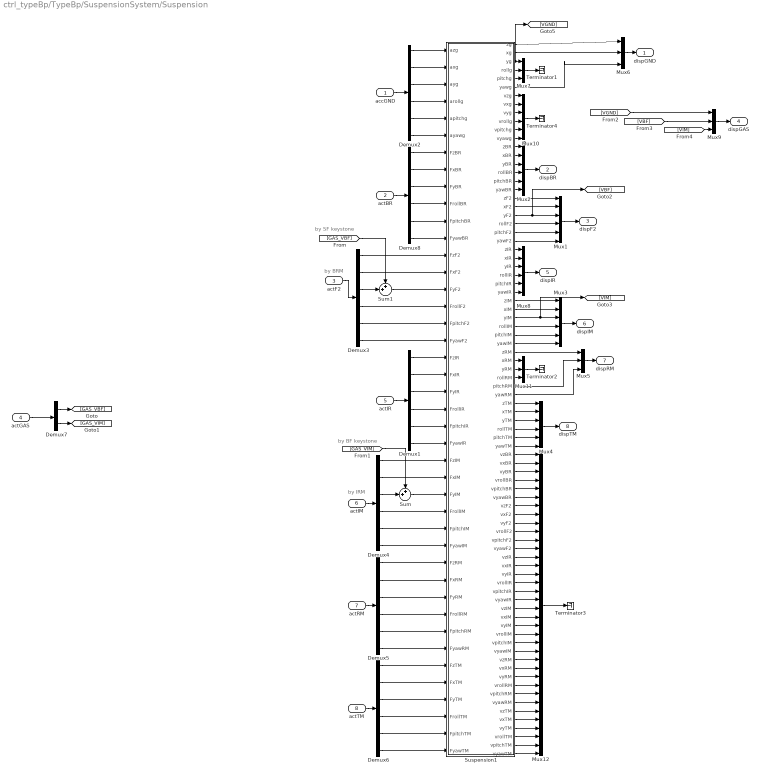
== system ctrl_typeBp/TypeBp/SuspensionSystem/Suspension ==
  note: by BF keystone
  note: by IRM
  note: by SF keystone
  note: by BRM
  accGND : Inport
  actBR : Inport  Port=2
  actF2 : Inport  Port=3
  actGAS : Inport  Port=4
  actIR : Inport  Port=5
  actIM : Inport  Port=6
  actRM : Inport  Port=7
  actTM : Inport  Port=8
  Demux{1..6,8} (7 alike) : Demux  Outputs=6
  Demux7 : Demux  Outputs=2
  Mux{1..4,8,10} (6 alike) : Mux  Inputs=6
  Mux{5..7,9,11} (5 alike) : Mux  Inputs=3
  Mux12 : Mux  Inputs=36
  Sum : Sum  Inputs=++|
  Sum1 : Sum  Inputs=++|
  Suspension1 : Subsystem
  Terminator{1..4} (4 alike) : Terminator
  dispGND : Outport
  dispBR : Outport  Port=2
  dispF2 : Outport  Port=3
  dispGAS : Outport  Port=4
  dispIR : Outport  Port=5
  dispIM : Outport  Port=6
  dispRM : Outport  Port=7
  dispTM : Outport  Port=8
  wires:
  Mux3/1 -> dispIM/1
  Mux8/1 -> dispIR/1
  Mux4/1 -> dispTM/1
  accGND/1 -> Demux2/1
  actTM/1 -> Demux6/1
  actIR/1 -> Demux1/1
  actRM/1 -> Demux5/1
  actIM/1 -> Demux4/1
  Mux5/1 -> dispRM/1
  Suspension1/31(zIM) -> Mux3/1
  Suspension1/32(xIM) -> Mux3/2
  Suspension1/34(rollIM) -> Mux3/4
  Suspension1/35(pitchIM) -> Mux3/5
  Suspension1/36(yawIM) -> Mux3/6
  Suspension1/25(zIR) -> Mux8/1
  Suspension1/26(xIR) -> Mux8/2
  Suspension1/27(yIR) -> Mux8/3
  Suspension1/28(rollIR) -> Mux8/4
  Suspension1/29(pitchIR) -> Mux8/5
  Suspension1/30(yawIR) -> Mux8/6
  Mux6/1 -> dispGND/1
  actGAS/1 -> Demux7/1
  actF2/1 -> Demux3/1
  Mux1/1 -> dispF2/1
  actBR/1 -> Demux8/1
  Demux4/3 -> Sum/2
  Mux2/1 -> dispBR/1
  Suspension1/33(yIM) -> [VIM], Mux3/3
  Mux9/1 -> dispGAS/1
  [VGND] -> Mux9/1
  Suspension1/37(zRM) -> Mux5/1
  Suspension1/41(pitchRM) -> Mux5/2
  Suspension1/42(yawRM) -> Mux5/3
  Suspension1/48(yawTM) -> Mux4/6
  Suspension1/43(zTM) -> Mux4/1
  Suspension1/46(rollTM) -> Mux4/4
  Suspension1/45(yTM) -> Mux4/3
  Suspension1/44(xTM) -> Mux4/2
  Suspension1/47(pitchTM) -> Mux4/5
  Demux3/3 -> Sum1/2
  [GAS_VBF] -> Sum1/1
  Demux7/1 -> [GAS_VBF]
  [GAS_VIM] -> Sum/1
  Demux7/2 -> [GAS_VIM]
  Mux7/1 -> Terminator1/1
  Mux10/1 -> Terminator4/1
  Demux2/2 -> Suspension1/2(axg)
  Demux2/4 -> Suspension1/4(arollg)
  Demux2/3 -> Suspension1/3(ayg)
  Demux2/6 -> Suspension1/6(ayawg)
  Demux2/5 -> Suspension1/5(apitchg)
  Demux2/1 -> Suspension1/1(azg)
  Demux8/6 -> Suspension1/12(FyawBR)
  Demux8/5 -> Suspension1/11(FpitchBR)
  Demux8/1 -> Suspension1/7(FzBR)
  Demux8/3 -> Suspension1/9(FyBR)
  Demux8/4 -> Suspension1/10(FrollBR)
  Demux8/2 -> Suspension1/8(FxBR)
  Demux3/2 -> Suspension1/14(FxF2)
  Demux3/1 -> Suspension1/13(FzF2)
  Sum1/1 -> Suspension1/15(FyF2)
  Demux3/4 -> Suspension1/16(FrollF2)
  Demux3/5 -> Suspension1/17(FpitchF2)
  Demux3/6 -> Suspension1/18(FyawF2)
  Demux1/5 -> Suspension1/23(FpitchIR)
  Demux1/3 -> Suspension1/21(FyIR)
  Demux1/4 -> Suspension1/22(FrollIR)
  Demux1/6 -> Suspension1/24(FyawIR)
  Demux1/1 -> Suspension1/19(FzIR)
  Demux1/2 -> Suspension1/20(FxIR)
  Demux4/1 -> Suspension1/25(FzIM)
  Demux4/2 -> Suspension1/26(FxIM)
  Sum/1 -> Suspension1/27(FyIM)
  Demux4/4 -> Suspension1/28(FrollIM)
  Demux4/5 -> Suspension1/29(FpitchIM)
  Demux4/6 -> Suspension1/30(FyawIM)
  Demux5/3 -> Suspension1/33(FyRM)
  Demux5/1 -> Suspension1/31(FzRM)
  Demux5/5 -> Suspension1/35(FpitchRM)
  Demux5/4 -> Suspension1/34(FrollRM)
  Demux5/2 -> Suspension1/32(FxRM)
  Demux5/6 -> Suspension1/36(FyawRM)
  Demux6/3 -> Suspension1/39(FyTM)
  Demux6/2 -> Suspension1/38(FxTM)
  Demux6/1 -> Suspension1/37(FzTM)
  Demux6/5 -> Suspension1/41(FpitchTM)
  Demux6/6 -> Suspension1/42(FyawTM)
  Demux6/4 -> Suspension1/40(FrollTM)
  Suspension1/1(zg) -> Mux6/1
  Suspension1/2(xg) -> Mux6/2
  Suspension1/6(yawg) -> Mux6/3
  Suspension1/3(yg) -> [VGND], Mux7/1
  Suspension1/4(rollg) -> Mux7/2
  Suspension1/5(pitchg) -> Mux7/3
  Suspension1/12(vyawg) -> Mux10/6
  Suspension1/10(vrollg) -> Mux10/4
  Suspension1/8(vxg) -> Mux10/2
  Suspension1/9(vyg) -> Mux10/3
  Suspension1/11(vpitchg) -> Mux10/5
  Suspension1/7(vzg) -> Mux10/1
  Suspension1/17(pitchBR) -> Mux2/5
  Suspension1/16(rollBR) -> Mux2/4
  Suspension1/15(yBR) -> Mux2/3
  Suspension1/18(yawBR) -> Mux2/6
  Suspension1/13(zBR) -> Mux2/1
  Suspension1/14(xBR) -> Mux2/2
  Suspension1/23(pitchF2) -> Mux1/5
  Suspension1/21(yF2) -> [VBF], Mux1/3
  Suspension1/24(yawF2) -> Mux1/6
  Suspension1/20(xF2) -> Mux1/2
  Suspension1/19(zF2) -> Mux1/1
  Suspension1/22(rollF2) -> Mux1/4
  [VBF] -> Mux9/2
  [VIM] -> Mux9/3
  Mux11/1 -> Terminator2/1
  Suspension1/38(xRM) -> Mux11/1
  Suspension1/39(yRM) -> Mux11/2
  Suspension1/40(rollRM) -> Mux11/3
  Mux12/1 -> Terminator3/1
  Suspension1/58(vrollF2) -> Mux12/10
  Suspension1/52(vrollBR) -> Mux12/4
  Suspension1/63(vyIR) -> Mux12/15
  Suspension1/65(vpitchIR) -> Mux12/17
  Suspension1/54(vyawBR) -> Mux12/6
  Suspension1/50(vxBR) -> Mux12/2
  Suspension1/62(vxIR) -> Mux12/14
  Suspension1/60(vyawF2) -> Mux12/12
  Suspension1/82(vrollTM) -> Mux12/34
  Suspension1/70(vrollIM) -> Mux12/22
  Suspension1/80(vxTM) -> Mux12/32
  Suspension1/72(vyawIM) -> Mux12/24
  Suspension1/79(vzTM) -> Mux12/31
  Suspension1/84(vyawTM) -> Mux12/36
  Suspension1/71(vpitchIM) -> Mux12/23
  Suspension1/75(vyRM) -> Mux12/27
  Suspension1/64(vrollIR) -> Mux12/16
  Suspension1/76(vrollRM) -> Mux12/28
  Suspension1/78(vyawRM) -> Mux12/30
  Suspension1/67(vzIM) -> Mux12/19
  Suspension1/81(vyTM) -> Mux12/33
  Suspension1/68(vxIM) -> Mux12/20
  Suspension1/83(vpitchTM) -> Mux12/35
  Suspension1/77(vpitchRM) -> Mux12/29
  Suspension1/74(vxRM) -> Mux12/26
  Suspension1/73(vzRM) -> Mux12/25
  Suspension1/69(vyIM) -> Mux12/21
  Suspension1/66(vyawIR) -> Mux12/18
  Suspension1/53(vpitchBR) -> Mux12/5
  Suspension1/55(vzF2) -> Mux12/7
  Suspension1/56(vxF2) -> Mux12/8
  Suspension1/61(vzIR) -> Mux12/13
  Suspension1/49(vzBR) -> Mux12/1
  Suspension1/59(vpitchF2) -> Mux12/11
  Suspension1/57(vyF2) -> Mux12/9
  Suspension1/51(vyBR) -> Mux12/3

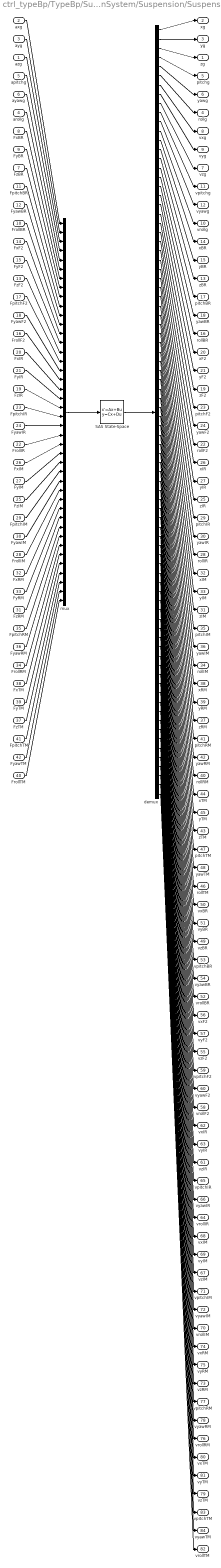
== system ctrl_typeBp/TypeBp/SuspensionSystem/Suspension/Suspension1 ==
  azg : Inport
  axg : Inport  Port=2
  ayg : Inport  Port=3
  arollg : Inport  Port=4
  apitchg : Inport  Port=5
  ayawg : Inport  Port=6
  FzBR : Inport  Port=7
  FxBR : Inport  Port=8
  FyBR : Inport  Port=9
  FrollBR : Inport  Port=10
  FpitchBR : Inport  Port=11
  FyawBR : Inport  Port=12
  FzF2 : Inport  Port=13
  FxF2 : Inport  Port=14
  FyF2 : Inport  Port=15
  FrollF2 : Inport  Port=16
  FpitchF2 : Inport  Port=17
  FyawF2 : Inport  Port=18
  FzIR : Inport  Port=19
  FxIR : Inport  Port=20
  FyIR : Inport  Port=21
  FrollIR : Inport  Port=22
  FpitchIR : Inport  Port=23
  FyawIR : Inport  Port=24
  FzIM : Inport  Port=25
  FxIM : Inport  Port=26
  FyIM : Inport  Port=27
  FrollIM : Inport  Port=28
  FpitchIM : Inport  Port=29
  FyawIM : Inport  Port=30
  FzRM : Inport  Port=31
  FxRM : Inport  Port=32
  FyRM : Inport  Port=33
  FrollRM : Inport  Port=34
  FpitchRM : Inport  Port=35
  FyawRM : Inport  Port=36
  FzTM : Inport  Port=37
  FxTM : Inport  Port=38
  FyTM : Inport  Port=39
  FrollTM : Inport  Port=40
  FpitchTM : Inport  Port=41
  FyawTM : Inport  Port=42
  SAS State-Space : StateSpace  A=sys1.A  B=sys1.B  C=sys1.C  D=sys1.D  X0=0  ContinuousStateAttributes='SUS_SS_MODEL'
  demux : Demux  Outputs=84
  mux : Mux  Inputs=42
  zg : Outport
  xg : Outport  Port=2
  yg : Outport  Port=3
  rollg : Outport  Port=4
  pitchg : Outport  Port=5
  yawg : Outport  Port=6
  vzg : Outport  Port=7
  vxg : Outport  Port=8
  vyg : Outport  Port=9
  vrollg : Outport  Port=10
  vpitchg : Outport  Port=11
  vyawg : Outport  Port=12
  zBR : Outport  Port=13
  xBR : Outport  Port=14
  yBR : Outport  Port=15
  rollBR : Outport  Port=16
  pitchBR : Outport  Port=17
  yawBR : Outport  Port=18
  zF2 : Outport  Port=19
  xF2 : Outport  Port=20
  yF2 : Outport  Port=21
  rollF2 : Outport  Port=22
  pitchF2 : Outport  Port=23
  yawF2 : Outport  Port=24
  zIR : Outport  Port=25
  xIR : Outport  Port=26
  yIR : Outport  Port=27
  rollIR : Outport  Port=28
  pitchIR : Outport  Port=29
  yawIR : Outport  Port=30
  zIM : Outport  Port=31
  xIM : Outport  Port=32
  yIM : Outport  Port=33
  rollIM : Outport  Port=34
  pitchIM : Outport  Port=35
  yawIM : Outport  Port=36
  zRM : Outport  Port=37
  xRM : Outport  Port=38
  yRM : Outport  Port=39
  rollRM : Outport  Port=40
  pitchRM : Outport  Port=41
  yawRM : Outport  Port=42
  zTM : Outport  Port=43
  xTM : Outport  Port=44
  yTM : Outport  Port=45
  rollTM : Outport  Port=46
  pitchTM : Outport  Port=47
  yawTM : Outport  Port=48
  vzBR : Outport  Port=49
  vxBR : Outport  Port=50
  vyBR : Outport  Port=51
  vrollBR : Outport  Port=52
  vpitchBR : Outport  Port=53
  vyawBR : Outport  Port=54
  vzF2 : Outport  Port=55
  vxF2 : Outport  Port=56
  vyF2 : Outport  Port=57
  vrollF2 : Outport  Port=58
  vpitchF2 : Outport  Port=59
  vyawF2 : Outport  Port=60
  vzIR : Outport  Port=61
  vxIR : Outport  Port=62
  vyIR : Outport  Port=63
  vrollIR : Outport  Port=64
  vpitchIR : Outport  Port=65
  vyawIR : Outport  Port=66
  vzIM : Outport  Port=67
  vxIM : Outport  Port=68
  vyIM : Outport  Port=69
  vrollIM : Outport  Port=70
  vpitchIM : Outport  Port=71
  vyawIM : Outport  Port=72
  vzRM : Outport  Port=73
  vxRM : Outport  Port=74
  vyRM : Outport  Port=75
  vrollRM : Outport  Port=76
  vpitchRM : Outport  Port=77
  vyawRM : Outport  Port=78
  vzTM : Outport  Port=79
  vxTM : Outport  Port=80
  vyTM : Outport  Port=81
  vrollTM : Outport  Port=82
  vpitchTM : Outport  Port=83
  vyawTM : Outport  Port=84
  wires:
  mux/1 -> SAS State-Space/1
  SAS State-Space/1 -> demux/1
  axg/1 -> mux/1
  ayg/1 -> mux/2
  azg/1 -> mux/3
  apitchg/1 -> mux/4
  ayawg/1 -> mux/5
  arollg/1 -> mux/6
  FxBR/1 -> mux/7
  FyBR/1 -> mux/8
  FzBR/1 -> mux/9
  FpitchBR/1 -> mux/10
  FyawBR/1 -> mux/11
  FrollBR/1 -> mux/12
  FxF2/1 -> mux/13
  FyF2/1 -> mux/14
  FzF2/1 -> mux/15
  FpitchF2/1 -> mux/16
  FyawF2/1 -> mux/17
  FrollF2/1 -> mux/18
  FxIR/1 -> mux/19
  FyIR/1 -> mux/20
  FzIR/1 -> mux/21
  FpitchIR/1 -> mux/22
  FyawIR/1 -> mux/23
  FrollIR/1 -> mux/24
  FxIM/1 -> mux/25
  FyIM/1 -> mux/26
  FzIM/1 -> mux/27
  FpitchIM/1 -> mux/28
  FyawIM/1 -> mux/29
  FrollIM/1 -> mux/30
  FxRM/1 -> mux/31
  FyRM/1 -> mux/32
  FzRM/1 -> mux/33
  FpitchRM/1 -> mux/34
  FyawRM/1 -> mux/35
  FrollRM/1 -> mux/36
  FxTM/1 -> mux/37
  FyTM/1 -> mux/38
  FzTM/1 -> mux/39
  FpitchTM/1 -> mux/40
  FyawTM/1 -> mux/41
  FrollTM/1 -> mux/42
  demux/1 -> xg/1
  demux/2 -> yg/1
  demux/3 -> zg/1
  demux/4 -> pitchg/1
  demux/5 -> yawg/1
  demux/6 -> rollg/1
  demux/7 -> vxg/1
  demux/8 -> vyg/1
  demux/9 -> vzg/1
  demux/10 -> vpitchg/1
  demux/11 -> vyawg/1
  demux/12 -> vrollg/1
  demux/13 -> xBR/1
  demux/14 -> yBR/1
  demux/15 -> zBR/1
  demux/16 -> pitchBR/1
  demux/17 -> yawBR/1
  demux/18 -> rollBR/1
  demux/19 -> xF2/1
  demux/20 -> yF2/1
  demux/21 -> zF2/1
  demux/22 -> pitchF2/1
  demux/23 -> yawF2/1
  demux/24 -> rollF2/1
  demux/25 -> xIR/1
  demux/26 -> yIR/1
  demux/27 -> zIR/1
  demux/28 -> pitchIR/1
  demux/29 -> yawIR/1
  demux/30 -> rollIR/1
  demux/31 -> xIM/1
  demux/32 -> yIM/1
  demux/33 -> zIM/1
  demux/34 -> pitchIM/1
  demux/35 -> yawIM/1
  demux/36 -> rollIM/1
  demux/37 -> xRM/1
  demux/38 -> yRM/1
  demux/39 -> zRM/1
  demux/40 -> pitchRM/1
  demux/41 -> yawRM/1
  demux/42 -> rollRM/1
  demux/43 -> xTM/1
  demux/44 -> yTM/1
  demux/45 -> zTM/1
  demux/46 -> pitchTM/1
  demux/47 -> yawTM/1
  demux/48 -> rollTM/1
  demux/49 -> vxBR/1
  demux/50 -> vyBR/1
  demux/51 -> vzBR/1
  demux/52 -> vpitchBR/1
  demux/53 -> vyawBR/1
  demux/54 -> vrollBR/1
  demux/55 -> vxF2/1
  demux/56 -> vyF2/1
  demux/57 -> vzF2/1
  demux/58 -> vpitchF2/1
  demux/59 -> vyawF2/1
  demux/60 -> vrollF2/1
  demux/61 -> vxIR/1
  demux/62 -> vyIR/1
  demux/63 -> vzIR/1
  demux/64 -> vpitchIR/1
  demux/65 -> vyawIR/1
  demux/66 -> vrollIR/1
  demux/67 -> vxIM/1
  demux/68 -> vyIM/1
  demux/69 -> vzIM/1
  demux/70 -> vpitchIM/1
  demux/71 -> vyawIM/1
  demux/72 -> vrollIM/1
  demux/73 -> vxRM/1
  demux/74 -> vyRM/1
  demux/75 -> vzRM/1
  demux/76 -> vpitchRM/1
  demux/77 -> vyawRM/1
  demux/78 -> vrollRM/1
  demux/79 -> vxTM/1
  demux/80 -> vyTM/1
  demux/81 -> vzTM/1
  demux/82 -> vpitchTM/1
  demux/83 -> vyawTM/1
  demux/84 -> vrollTM/1
